simulink model "fun"  (R2014a)
settings: Solver=ode45  StartTime=0.0  StopTime=10.0  RelTol=1e-3
libraries: fl_lib x6, elec_lib x1
settings Model: Creator=SKY  LastModifiedBy=SKY

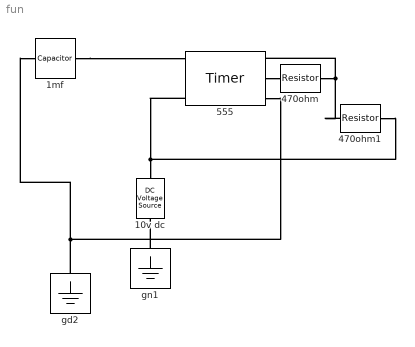
== system fun ==
  10v dc : fl_lib/Electrical/Electrical Sources/DC Voltage Source  v0=10 V
  1mf : fl_lib/Electrical/Electrical Elements/Capacitor  c=1e-3 F  r=1e-6 Ohm  g=0 1/Ohm  i_specify=off  i_priority=High  i=0 A  v_specify=off  v_priority=High  v=0 V  vc_specify=off  vc_priority=High  vc=0 V
  470ohm : fl_lib/Electrical/Electrical Elements/Resistor  R=470 Ohm  i_specify=off  i_priority=High  i=0 A  v_specify=off  v_priority=High  v=0 V
  470ohm1 : fl_lib/Electrical/Electrical Elements/Resistor  R=470 Ohm  i_specify=off  i_priority=High  i=0 A  v_specify=off  v_priority=High  v=0 V
  555 : elec_lib/Integrated Circuits/Timer  V_CC=15 V  V_OL=0 V  V_OH=14.1 V  R_OUT=8 Ohm  Delay=1e-7 s  R_DIV=5 kOhm  R_closed=12 Ohm  R_open=5e+8 Ohm
  gd2 : fl_lib/Electrical/Electrical Elements/Electrical Reference
  gn1 : fl_lib/Electrical/Electrical Elements/Electrical Reference
  connections:
  555/LConn3 -- 470ohm1/RConn1 -- 10v dc/LConn1
  gn1/LConn1 -- 10v dc/RConn1
  gd2/LConn1 -- 555/RConn3 -- 1mf/LConn1
  555/RConn2 -- 470ohm/LConn1
  470ohm/RConn1 -- 555/RConn1 -- 470ohm1/LConn1
  1mf/RConn1 -- 555/LConn1
